simulink subsystem "iPoC"  (R2022b)
settings: Solver=VariableStepAuto  StartTime=0.0  StopTime=10.0  RelTol=1e-3
values from neighbouring files (symbols this model uses):
  d = 1    [IPoC_setup.m]
  g = -10    [IPoC_setup.m]
  L = 0.2    [IPoC_setup.m]
  m = 0.05    [IPoC_setup.m]
  M = 0.20    (= 0.2)    [IPoC_setup.m]
  x0 = [0, pi, 0]'    [IPoC_setup.m]
undefined symbols (not defined in the file or in its folder): DiscIntNeverNeededParam
settings Model: Creator=Benja  LastModifiedBy=Benja

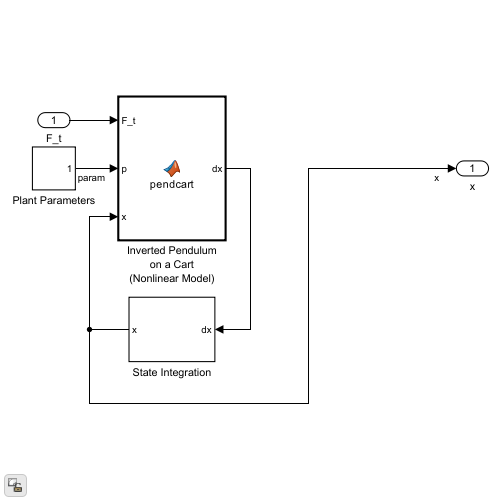
[thumbnail: Simulink's stored preview of the top-level diagram]
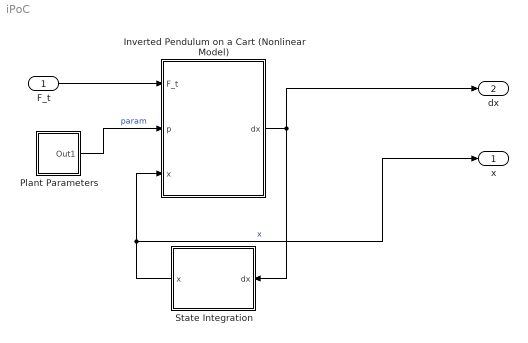
== system iPoC ==
  F_t : Inport
  Inverted Pendulum on a Cart (Nonlinear Model) : MATLAB Function  TreatAsAtomicUnit=on
  Plant Parameters : Subsystem
  State Integration : Subsystem
  x : Outport  PortDimensions=[3,1]
  dx : Outport  Port=2  PortDimensions=[3,1]
  wires:
  State Integration/1(x) -> x/1, Inverted Pendulum on a Cart (Nonlinear Model)/3(x)  "x"
  F_t/1 -> Inverted Pendulum on a Cart (Nonlinear Model)/1(F_t)
  Plant Parameters/1(Out1) -> Inverted Pendulum on a Cart (Nonlinear Model)/2(p)  "param"
  Inverted Pendulum on a Cart (Nonlinear Model)/1(dx) -> State Integration/1(dx), dx/1

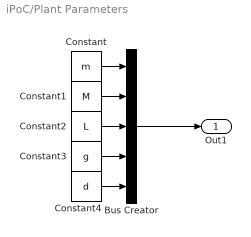
== system iPoC/Plant Parameters ==
  Bus Creator : BusCreator  Inputs=5
  Constant : Constant  Value=m
  Constant1 : Constant  Value=M
  Constant2 : Constant  Value=L
  Constant3 : Constant  Value=g
  Constant4 : Constant  Value=d
  Out1 : Outport
  wires:
  Constant/1 -> Bus Creator/1
  Constant1/1 -> Bus Creator/2
  Constant2/1 -> Bus Creator/3
  Bus Creator/1 -> Out1/1
  Constant3/1 -> Bus Creator/4
  Constant4/1 -> Bus Creator/5

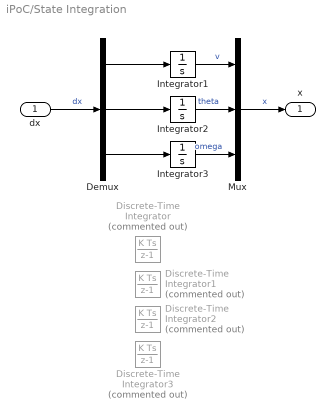
== system iPoC/State Integration ==
  dx : Inport
  Demux : Demux  Outputs=3
  Discrete-Time Integrator : DiscreteIntegrator  Commented=on  InitialCondition=x0(1)  SampleTime=-1  ICPrevOutput=DiscIntNeverNeededParam  ICPrevScaledInput=DiscIntNeverNeededParam
  Discrete-Time Integrator1 : DiscreteIntegrator  Commented=on  InitialCondition=x0(2)  SampleTime=-1  ICPrevOutput=DiscIntNeverNeededParam  ICPrevScaledInput=DiscIntNeverNeededParam
  Discrete-Time Integrator2 : DiscreteIntegrator  Commented=on  InitialCondition=x0(3)  SampleTime=-1  ICPrevOutput=DiscIntNeverNeededParam  ICPrevScaledInput=DiscIntNeverNeededParam
  Discrete-Time Integrator3 : DiscreteIntegrator  Commented=on  InitialCondition=x0(4)  SampleTime=-1  ICPrevOutput=DiscIntNeverNeededParam  ICPrevScaledInput=DiscIntNeverNeededParam
  Integrator1 : Integrator  InitialCondition=x0(1)  ContinuousStateAttributes='vel'
  Integrator2 : Integrator  InitialCondition=x0(2)  ContinuousStateAttributes='theta'
  Integrator3 : Integrator  InitialCondition=x0(3)  ContinuousStateAttributes='omega'
  Mux : Mux  Inputs=3
  x : Outport
  wires:
  Demux/1 -> Integrator1/1
  Integrator1/1 -> Mux/1  "v"
  Integrator2/1 -> Mux/2  "theta"
  Demux/3 -> Integrator3/1
  Demux/2 -> Integrator2/1
  Integrator3/1 -> Mux/3  "omega"
  Mux/1 -> x/1  "x"
  dx/1 -> Demux/1  "dx"

== matlab function iPoC/Inverted Pendulum on a Cart (Nonlinear Model) ==
  data: F_t input; p input; x input; dx output
%% Inverted Pendulum
% Taken from Brunton, Kutz - Data Driven Science and Engineering, p. 301
function dx = pendcart(F_t,p, x) 
% Parameter Reading
m = p(1);
M = p(2);
L = p(3);
g = p(4);
d = p(5);

% Preallocation
dx = zeros(3,1);
x = zeros(3,1);

% Trigonometric Functions
Sx = sin(x(2,1)); 
Cx = cos(x(2,1));
D = m*L*L*(M+m*(1-Cx^2)); % Divider

% State derivative 
% dx(1,1) = x(2); % dx
dx(1,1) = (1/D)*(-m^2*L^2*g*Cx*Sx + m*L^2*(m*L*x(3,1)^2*Sx - d*x(1,1))) + m*L*L*(1/D)*F_t; % dv
dx(2,1) = x(3,1); % dtheta
dx(3,1) = (1/D)*((m+M)*m*g*L*Sx - m*L*Cx*(m*L*x(3,1)^2*Sx - d*x(1,1))) - m*L*Cx*(1/D)*F_t; % domega
